simulink model "clrrtsf"  (R2020a)
settings: Solver=FixedStepAuto  StartTime=0.0  StopTime=inf  FixedStep=0.2  RelTol=1e-3
model workspace (MAT data in the model file):
  IC_theta0 = Simulink.Signal
  IC_theta0.DataType = 'auto'
  IC_theta0.Dimensions = -1
  IC_theta0.DimensionsMode = 'auto'
  IC_theta0.Complexity = 'auto'
  IC_theta0.SampleTime = -1
  IC_theta0.SamplingMode = 'auto'
  IC_theta0.InitialValue = '0'
  IC_x0 = Simulink.Signal
  IC_x0.DataType = 'auto'
  IC_x0.Dimensions = -1
  IC_x0.DimensionsMode = 'auto'
  IC_x0.Complexity = 'auto'
  IC_x0.SampleTime = -1
  IC_x0.SamplingMode = 'auto'
  IC_x0.InitialValue = '0'
  IC_x1 = Simulink.Signal
  IC_x1.DataType = 'auto'
  IC_x1.Dimensions = -1
  IC_x1.DimensionsMode = 'auto'
  IC_x1.Complexity = 'auto'
  IC_x1.SampleTime = -1
  IC_x1.SamplingMode = 'auto'
  IC_x1.InitialValue = '0'
  IC_y0 = Simulink.Signal
  IC_y0.DataType = 'auto'
  IC_y0.Dimensions = -1
  IC_y0.DimensionsMode = 'auto'
  IC_y0.Complexity = 'auto'
  IC_y0.SampleTime = -1
  IC_y0.SamplingMode = 'auto'
  IC_y1 = Simulink.Signal
  IC_y1.DataType = 'auto'
  IC_y1.Dimensions = -1
  IC_y1.DimensionsMode = 'auto'
  IC_y1.Complexity = 'auto'
  IC_y1.SampleTime = -1
  IC_y1.SamplingMode = 'auto'
  IC_y1.InitialValue = '0'
  contsim_time = Simulink.Signal
  contsim_time.DataType = 'double'
  contsim_time.Dimensions = [1 1]
  contsim_time.DimensionsMode = 'auto'
  contsim_time.Complexity = 'real'
  contsim_time.SampleTime = -1
  contsim_time.SamplingMode = 'auto'
  indicator = Simulink.Signal
  indicator.DataType = 'double'
  indicator.Dimensions = [1 4]
  indicator.DimensionsMode = 'auto'
  indicator.Complexity = 'real'
  indicator.SampleTime = -1
  indicator.SamplingMode = 'auto'
  indicator.InitialValue = '[0 0]'
  ip = Simulink.Signal
  ip.DataType = 'double'
  ip.Dimensions = [1 2]
  ip.DimensionsMode = 'auto'
  ip.Complexity = 'real'
  ip.SampleTime = -1
  ip.SamplingMode = 'auto'
  szxx1 = Simulink.Signal
  szxx1.DataType = 'double'
  szxx1.Dimensions = [1 1]
  szxx1.DimensionsMode = 'auto'
  szxx1.Complexity = 'real'
  szxx1.SampleTime = -1
  szxx1.SamplingMode = 'auto'
  szxx1.InitialValue = '0'
values from neighbouring files (symbols this model uses):
  indsimtime = 150    [clrrtsf_Initializ.m]
  L_0b = 0.48    [clrrtsf_Initializ.m]    (also in clrrtsolutionplot.m)
  L_0f = 3.8    [clrrtsf_Initializ.m]    (also in clrrtsolutionplot.m)
  L_1f = 7.21    [clrrtsf_Initializ.m]    (also in clrrtsolutionplot.m)
  LD = 10    [clrrtsf_Initializ.m]
  pinit = [80 160 pi 0]    [clrrtsf_Initializ.m]
  tn = zeros(N,14)    [clrrtsf_Initializ.m]    (also in clrrtsolutionplot.m = out.tree)
  veh_path = zeros(indsimtime,6)    [clrrtsf_Initializ.m]
  veh_path_col = zeros(indsimtime,6,N)    [clrrtsf_Initializ.m]
  xx = [-50:0.5:50]'    [clrrtsf_Initializ.m]
  yy = [-50:0.5:50]'    [clrrtsf_Initializ.m]
  Zf = griddata(x,y,znew,xnewt,ynewt)    [clrrtsf_Initializ.m]
  Zr = griddata(x,y,znewr,xnewt,ynewt)    [clrrtsf_Initializ.m]
undefined symbols (not defined in the file or in its folder): DiscIntNeverNeededParam, IC_theta1
libraries: simulink x1
(part 1 of 2)
settings Model: PauseTimes=0  OrderedModelArguments=off  Creator=giridhar  LastModifiedBy=giridhar
settings SolverCC: AlgebraicLoopSolver=LineSearch  MinimalZcImpactIntegration=on
settings DebuggingCC: ReadBeforeWriteMsg=DisableAll  WriteAfterWriteMsg=DisableAll  WriteAfterReadMsg=DisableAll  MultiTaskDSMMsg=none  SFUnusedDataAndEventsDiag=none  UnderSpecifiedDimensionMsg=warning
settings ModelReferenceCC: UpdateModelReferenceTargets=IfOutOfDate
settings SFSimCC: SFSimEcho=off

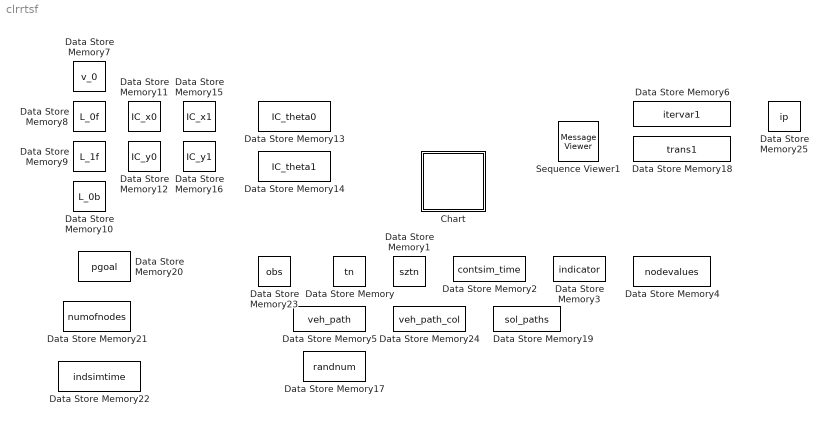
== system clrrtsf ==
  Chart : Stateflow chart  TreatAsAtomicUnit=on
  Data Store Memory : DataStoreMemory  DataStoreName=tn  ReadBeforeWriteMsg=warning  WriteAfterWriteMsg=warning  WriteAfterReadMsg=warning  InitialValue=tn  VectorParams1D=off  ShowAdditionalParam=off  OutDataTypeStr=double
  Data Store Memory1 : DataStoreMemory  DataStoreName=sztn  ReadBeforeWriteMsg=warning  WriteAfterWriteMsg=warning  WriteAfterReadMsg=warning  InitialValue=sztn  ShowAdditionalParam=off  OutDataTypeStr=double
  Data Store Memory10 : DataStoreMemory  DataStoreName=L_0b  ReadBeforeWriteMsg=warning  WriteAfterWriteMsg=warning  WriteAfterReadMsg=warning  InitialValue=0.48  VectorParams1D=off  ShowAdditionalParam=off  OutDataTypeStr=double  Dimensions=[1 1]
  Data Store Memory11 : DataStoreMemory  DataStoreName=IC_x0  ReadBeforeWriteMsg=warning  WriteAfterWriteMsg=warning  WriteAfterReadMsg=warning  VectorParams1D=off  ShowAdditionalParam=off  OutDataTypeStr=double  Dimensions=[1 1]
  Data Store Memory12 : DataStoreMemory  DataStoreName=IC_y0  ReadBeforeWriteMsg=warning  WriteAfterWriteMsg=warning  WriteAfterReadMsg=warning  VectorParams1D=off  ShowAdditionalParam=off  OutDataTypeStr=double  Dimensions=[1 1]
  Data Store Memory13 : DataStoreMemory  DataStoreName=IC_theta0  ReadBeforeWriteMsg=warning  WriteAfterWriteMsg=warning  WriteAfterReadMsg=warning  VectorParams1D=off  ShowAdditionalParam=off  OutDataTypeStr=double  Dimensions=[1 1]
  Data Store Memory14 : DataStoreMemory  DataStoreName=IC_theta1  ReadBeforeWriteMsg=warning  WriteAfterWriteMsg=warning  WriteAfterReadMsg=warning  VectorParams1D=off  ShowAdditionalParam=off  OutDataTypeStr=double  Dimensions=[1 1]
  Data Store Memory15 : DataStoreMemory  DataStoreName=IC_x1  ReadBeforeWriteMsg=warning  WriteAfterWriteMsg=warning  WriteAfterReadMsg=warning  VectorParams1D=off  ShowAdditionalParam=off  OutDataTypeStr=double  Dimensions=[1 1]  StateMustResolveToSignalObject=on
  Data Store Memory16 : DataStoreMemory  DataStoreName=IC_y1  ReadBeforeWriteMsg=warning  WriteAfterWriteMsg=warning  WriteAfterReadMsg=warning  VectorParams1D=off  ShowAdditionalParam=off  OutDataTypeStr=double  Dimensions=[1 1]  StateMustResolveToSignalObject=on
  Data Store Memory17 : DataStoreMemory  DataStoreName=randnum  ReadBeforeWriteMsg=warning  WriteAfterWriteMsg=warning  WriteAfterReadMsg=warning  InitialValue=randnum  ShowAdditionalParam=off  OutDataTypeStr=double
  Data Store Memory18 : DataStoreMemory  DataStoreName=trans1  ReadBeforeWriteMsg=warning  WriteAfterWriteMsg=warning  WriteAfterReadMsg=warning  VectorParams1D=off  ShowAdditionalParam=off  OutDataTypeStr=double
  Data Store Memory19 : DataStoreMemory  DataStoreName=sol_paths  ReadBeforeWriteMsg=warning  WriteAfterWriteMsg=warning  WriteAfterReadMsg=warning  ShowAdditionalParam=off
  Data Store Memory2 : DataStoreMemory  DataStoreName=contsim_time  ReadBeforeWriteMsg=warning  WriteAfterWriteMsg=warning  WriteAfterReadMsg=warning  VectorParams1D=off  ShowAdditionalParam=off  OutDataTypeStr=double  Dimensions=[1 1]  StateMustResolveToSignalObject=on
  Data Store Memory20 : DataStoreMemory  DataStoreName=pgoal  ReadBeforeWriteMsg=warning  WriteAfterWriteMsg=warning  WriteAfterReadMsg=warning  InitialValue=pgoal  VectorParams1D=off  ShowAdditionalParam=off  OutDataTypeStr=double
  Data Store Memory21 : DataStoreMemory  DataStoreName=numofnodes  ReadBeforeWriteMsg=warning  WriteAfterWriteMsg=warning  WriteAfterReadMsg=warning  InitialValue=numofnodes  VectorParams1D=off  ShowAdditionalParam=off  OutDataTypeStr=double
  Data Store Memory22 : DataStoreMemory  DataStoreName=indsimtime  ReadBeforeWriteMsg=warning  WriteAfterWriteMsg=warning  WriteAfterReadMsg=warning  InitialValue=indsimtime  ShowAdditionalParam=off  OutDataTypeStr=double
  Data Store Memory23 : DataStoreMemory  DataStoreName=obs  ReadBeforeWriteMsg=warning  WriteAfterWriteMsg=warning  WriteAfterReadMsg=warning  InitialValue=obs  VectorParams1D=off  ShowAdditionalParam=off  OutDataTypeStr=double
  Data Store Memory24 : DataStoreMemory  DataStoreName=veh_path_col  ReadBeforeWriteMsg=warning  WriteAfterWriteMsg=warning  WriteAfterReadMsg=warning  InitialValue=veh_path_col  VectorParams1D=off  ShowAdditionalParam=off  OutDataTypeStr=double
  Data Store Memory25 : DataStoreMemory  DataStoreName=ip  ReadBeforeWriteMsg=warning  WriteAfterWriteMsg=warning  WriteAfterReadMsg=warning  InitialValue=[0 0]  VectorParams1D=off  ShowAdditionalParam=off  OutDataTypeStr=double  Dimensions=[1 2]  StateMustResolveToSignalObject=on
  Data Store Memory3 : DataStoreMemory  DataStoreName=indicator  ReadBeforeWriteMsg=warning  WriteAfterWriteMsg=warning  WriteAfterReadMsg=warning  InitialValue=[0 0 0 0]  VectorParams1D=off  ShowAdditionalParam=off  OutDataTypeStr=double
  Data Store Memory4 : DataStoreMemory  DataStoreName=nodevalues  ReadBeforeWriteMsg=warning  WriteAfterWriteMsg=warning  WriteAfterReadMsg=warning  InitialValue=[0 0 0 0 0 0 0 0]  VectorParams1D=off  ShowAdditionalParam=off  OutDataTypeStr=double  Dimensions=[1 8]
  Data Store Memory5 : DataStoreMemory  DataStoreName=veh_path  ReadBeforeWriteMsg=warning  WriteAfterWriteMsg=warning  WriteAfterReadMsg=warning  InitialValue=veh_path  VectorParams1D=off  ShowAdditionalParam=off  OutDataTypeStr=double
  Data Store Memory6 : DataStoreMemory  DataStoreName=itervar1  ReadBeforeWriteMsg=warning  WriteAfterWriteMsg=warning  WriteAfterReadMsg=warning  VectorParams1D=off  ShowAdditionalParam=off  OutDataTypeStr=double
  Data Store Memory7 : DataStoreMemory  DataStoreName=v_0  ReadBeforeWriteMsg=warning  WriteAfterWriteMsg=warning  WriteAfterReadMsg=warning  InitialValue=v_0  VectorParams1D=off  ShowAdditionalParam=off  OutDataTypeStr=double  Dimensions=[1 1]
  Data Store Memory8 : DataStoreMemory  DataStoreName=L_0f  ReadBeforeWriteMsg=warning  WriteAfterWriteMsg=warning  WriteAfterReadMsg=warning  InitialValue=3.8  VectorParams1D=off  ShowAdditionalParam=off  OutDataTypeStr=double  Dimensions=[1 1]
  Data Store Memory9 : DataStoreMemory  DataStoreName=L_1f  ReadBeforeWriteMsg=warning  WriteAfterWriteMsg=warning  WriteAfterReadMsg=warning  InitialValue=7.21  VectorParams1D=off  ShowAdditionalParam=off  OutDataTypeStr=double  Dimensions=[1 1]
  Sequence Viewer1 : MessageViewer  History=1000  SavedRootId=#

== system clrrtsf/Chart/costcalculation.costcal ==
  i : Inport  OutDataTypeStr=double  PortDimensions=[1 1]
  f : TriggerPort  TriggerType=function-call  VariantControl=(inherit)
      settings: CopyFcn=Stateflow.SLINSF.SimulinkMan.removeBlockPreDeleteFcn  PreDeleteFcn=Stateflow.SLINSF.SimulinkMan.unsafePredeleteFcn
  Add : Sum
  Assignment5 : Assignment  NumberOfDimensions=2  DiagnosticForDimensions=Warning  IndexOptions=Index vector (port),Index vector (dialog)  Indices=1,1  OutputSizes=1,1
  Constant : Constant
  Data Store Read : DataStoreRead  DataStoreName=veh_path
  Data Store Read1 : DataStoreRead  DataStoreName=tn  DataStoreElements=tn(:,6)
  Data Store Write : DataStoreWrite  DataStoreName=tn  DataStoreElements=tn(:,6)
  MATLAB Function : MATLAB Function  TreatAsAtomicUnit=on
  wires:
  Data Store Read/1 -> MATLAB Function/1(veh_path)
  MATLAB Function/1(costt) -> Assignment5/2
  Data Store Read1/1 -> Assignment5/1
  Assignment5/1 -> Data Store Write/1
  i/1 -> Add/1
  Add/1 -> Assignment5/3
  Constant/1 -> Add/2

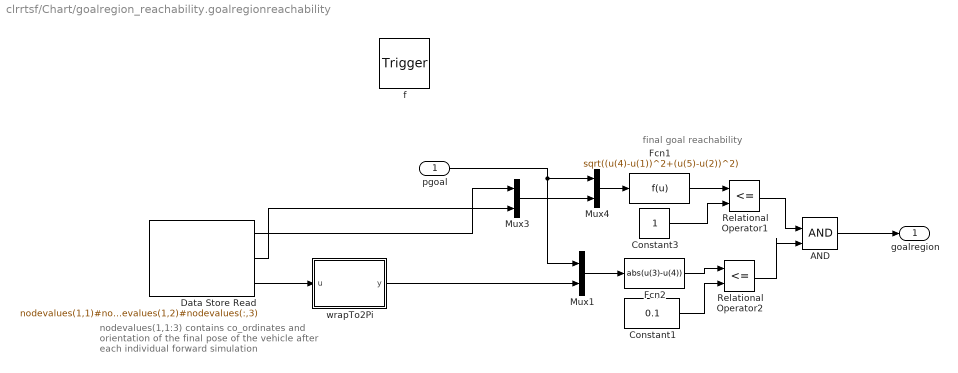
== system clrrtsf/Chart/goalregion_reachability.goalregionreachability ==
  note: nodevalues(1,1:3) contains co_ordinates
      | and orientation of the final pose of the
      | vehicle after each individual forward simulation
  note: final goal reachability
  pgoal : Inport  OutDataTypeStr=double  PortDimensions=[1 3]
  f : TriggerPort  TriggerType=function-call  VariantControl=(inherit)
      settings: CopyFcn=Stateflow.SLINSF.SimulinkMan.removeBlockPreDeleteFcn  PreDeleteFcn=Stateflow.SLINSF.SimulinkMan.unsafePredeleteFcn
  AND : Logic  IconShape=distinctive  AllPortsSameDT=off  OutDataTypeStr=boolean
  Constant1 : Constant  Value=0.1
  Constant3 : Constant
  Data Store Read : DataStoreRead  DataStoreName=nodevalues  DataStoreElements=nodevalues(1,1)#nodevalues(1,2)#nodevalues(:,3)
  Fcn1 : Fcn  Expr=sqrt((u(4)-u(1))^2+(u(5)-u(2))^2)
  Fcn2 : Fcn  Expr=abs(u(3)-u(4))
  Mux1 : Mux  Inputs=2
  Mux3 : Mux  Inputs=2
  Mux4 : Mux  Inputs=2
  Relational Operator1 : RelationalOperator  Operator=<=  OutDataTypeStr=boolean  RndMeth=Simplest
  Relational Operator2 : RelationalOperator  Operator=<=  OutDataTypeStr=boolean  RndMeth=Simplest
  wrapTo2Pi : MATLAB Function  TreatAsAtomicUnit=on
  goalregion : Outport
  wires:
  Constant1/1 -> Relational Operator2/2
  Relational Operator2/1 -> AND/2
  Mux1/1 -> Fcn2/1
  pgoal/1 -> Mux4/1, Mux1/1
  Mux3/1 -> Mux4/2
  Fcn2/1 -> Relational Operator2/1
  Constant3/1 -> Relational Operator1/2
  Fcn1/1 -> Relational Operator1/1
  Mux4/1 -> Fcn1/1
  Relational Operator1/1 -> AND/1
  Data Store Read/1 -> Mux3/1
  Data Store Read/2 -> Mux3/2
  Data Store Read/3 -> wrapTo2Pi/1(u)
  AND/1 -> goalregion/1
  wrapTo2Pi/1(y) -> Mux1/2

== system clrrtsf/Chart/output_to_workspace.output1wpace ==
  note: output to matlab workspace, all the details related to planning tree
      |  which were stored in the datastore "tn"
  note: output to matlab workspace, all the path co_ordinates and orientationof vehicle
      |  which were stored in the datastore "veh_path_col"
  f : TriggerPort  TriggerType=function-call  VariantControl=(inherit)
      settings: CopyFcn=Stateflow.SLINSF.SimulinkMan.removeBlockPreDeleteFcn  PreDeleteFcn=Stateflow.SLINSF.SimulinkMan.unsafePredeleteFcn
  Data Store Read : DataStoreRead  DataStoreName=tn  DataStoreElements=tn(:,:)
  Data Store Read1 : DataStoreRead  DataStoreName=veh_path_col  DataStoreElements=veh_path_col(:,1:4,:)
  To Workspace : ToWorkspace  VariableName=veh_path_col  SampleTime=-1
  To Workspace1 : ToWorkspace  VariableName=tree  SampleTime=-1
  wires:
  Data Store Read/1 -> To Workspace1/1
  Data Store Read1/1 -> To Workspace/1

== system clrrtsf/Chart/propagateorForwardsimulationstage.propagate ==
  note: subsystem to update
      | current start point node
      | and resets variables
      |  "itervar1" and "trans1"
  note: tractor longitudinal velocity
  note: gp is the intermediate goal point for the current
      | forward simulation, it can be a random sample
      | or a goal sample
  note: Nn_ is the node number of current start point, selected
      | based on the nearest neighbour or cheapest neighbour strategy
      | is uded to index into tree to find respective co-ordinates
  v_0 : Inport  OutDataTypeStr=double  PortDimensions=1
  gp : Inport  Port=2  OutMin=1  OutMax=2  OutDataTypeStr=double  PortDimensions=[1 3]
  Nn_ : Inport  Port=3  OutDataTypeStr=double  PortDimensions=1
  g : TriggerPort  TriggerType=function-call  VariantControl=(inherit)  SampleTime=0.2
      settings: CopyFcn=Stateflow.SLINSF.SimulinkMan.removeBlockPreDeleteFcn  PreDeleteFcn=Stateflow.SLINSF.SimulinkMan.unsafePredeleteFcn
  Data Store Read : DataStoreRead  DataStoreName=itervar1
  Delay : Delay  DelayLength=1
  Enabled Subsystem : Subsystem  TreatAsAtomicUnit=on
  Resettable Subsystem : Subsystem  Priority=1  TreatAsAtomicUnit=on
  Subsystem : Subsystem  Priority=2
  wires:
  gp/1 -> Subsystem/2(gp), Resettable Subsystem/2(gp)
  v_0/1 -> Resettable Subsystem/1(v_0)
  Nn_/1 -> Resettable Subsystem/3(Nn_), Enabled Subsystem/1(Nn_)
  Data Store Read/1 -> Subsystem/Enable, Subsystem/1(In1), Delay/1
  Delay/1 -> Enabled Subsystem/Enable, Resettable Subsystem/Reset

== system clrrtsf/Chart/stage1.f ==
  note: nearest neighbour
  sr : Inport  OutDataTypeStr=double  PortDimensions=[1 2]
  i : Inport  Port=2  OutDataTypeStr=double  PortDimensions=1
  f : TriggerPort  TriggerType=function-call  VariantControl=(inherit)  SampleTime=0.2
      settings: CopyFcn=Stateflow.SLINSF.SimulinkMan.removeBlockPreDeleteFcn  PreDeleteFcn=Stateflow.SLINSF.SimulinkMan.unsafePredeleteFcn
  For Iterator Subsystem : Subsystem  TreatAsAtomicUnit=on
  Nn : Outport  OutDataTypeStr=double
  wires:
  sr/1 -> For Iterator Subsystem/1(sr)
  For Iterator Subsystem/1(Nn) -> Nn/1
  i/1 -> For Iterator Subsystem/2(i)

== system clrrtsf/Chart/stage1.f_ ==
  note: cheapest neighbour
  note: random sample
  sr : Inport  OutDataTypeStr=double  PortDimensions=[1 2]
  i : Inport  Port=2  OutDataTypeStr=double  PortDimensions=1
  f : TriggerPort  TriggerType=function-call  VariantControl=(inherit)  SampleTime=0.2
      settings: CopyFcn=Stateflow.SLINSF.SimulinkMan.removeBlockPreDeleteFcn  PreDeleteFcn=Stateflow.SLINSF.SimulinkMan.unsafePredeleteFcn
  For Iterator Subsystem : Subsystem  TreatAsAtomicUnit=on
  Nn : Outport  OutDataTypeStr=double
  wires:
  sr/1 -> For Iterator Subsystem/1(sr)
  For Iterator Subsystem/1(Nn) -> Nn/1
  i/1 -> For Iterator Subsystem/2(i)

== system clrrtsf/Chart/stopsimulation ==
  Action Port : ActionPort
      settings: CopyFcn=Stateflow.SLINSF.SimulinkMan.removeBlockPreDeleteFcn  PreDeleteFcn=Stateflow.SLINSF.SimulinkMan.unsafePredeleteFcn
  Constant : Constant
  Stop Simulation : Stop
  wires:
  Constant/1 -> Stop Simulation/1

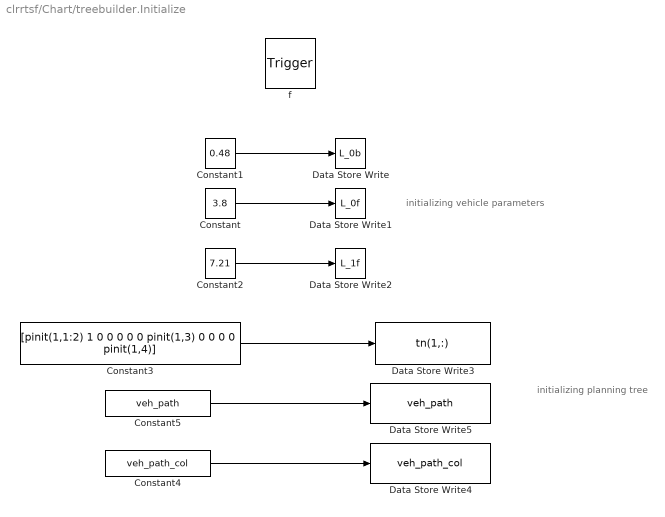
== system clrrtsf/Chart/treebuilder.Initialize ==
  note: initializing vehicle parameters
  note: initializing planning tree
  f : TriggerPort  TriggerType=function-call  VariantControl=(inherit)
      settings: CopyFcn=Stateflow.SLINSF.SimulinkMan.removeBlockPreDeleteFcn  PreDeleteFcn=Stateflow.SLINSF.SimulinkMan.unsafePredeleteFcn
  Constant : Constant  Value=3.8  VectorParams1D=off
  Constant1 : Constant  Value=0.48  VectorParams1D=off
  Constant2 : Constant  Value=7.21  VectorParams1D=off
  Constant3 : Constant  Value=[pinit(1,1:2) 1 0 0 0 0 0 pinit(1,3) 0 0 0 0 pinit(1,4)]  VectorParams1D=off
  Constant4 : Constant  Value=veh_path_col  VectorParams1D=off
  Constant5 : Constant  Value=veh_path  VectorParams1D=off
  Data Store Write : DataStoreWrite  DataStoreName=L_0b
  Data Store Write1 : DataStoreWrite  DataStoreName=L_0f
  Data Store Write2 : DataStoreWrite  DataStoreName=L_1f
  Data Store Write3 : DataStoreWrite  DataStoreName=tn  DataStoreElements=tn(1,:)
  Data Store Write4 : DataStoreWrite  DataStoreName=veh_path_col
  Data Store Write5 : DataStoreWrite  DataStoreName=veh_path
  wires:
  Constant/1 -> Data Store Write1/1
  Constant2/1 -> Data Store Write2/1
  Constant1/1 -> Data Store Write/1
  Constant3/1 -> Data Store Write3/1
  Constant4/1 -> Data Store Write4/1
  Constant5/1 -> Data Store Write5/1

== system clrrtsf/Chart/treebuilder.cumilativecost ==
  "i " : Inport  OutDataTypeStr=double  PortDimensions=[1 1]
  f : TriggerPort  TriggerType=function-call  VariantControl=(inherit)
      settings: CopyFcn=Stateflow.SLINSF.SimulinkMan.removeBlockPreDeleteFcn  PreDeleteFcn=Stateflow.SLINSF.SimulinkMan.unsafePredeleteFcn
  Assignment6 : Assignment  NumberOfDimensions=2  DiagnosticForDimensions=Warning  IndexOptions=Index vector (port),Index vector (dialog)  Indices=1,1  OutputSizes=1,1
  Data Store Read : DataStoreRead  DataStoreName=tn
  Data Store Read1 : DataStoreRead  DataStoreName=tn  DataStoreElements=tn(:,7)
  Data Store Write : DataStoreWrite  DataStoreName=tn  DataStoreElements=tn(:,7)
  MATLAB Function : MATLAB Function  TreatAsAtomicUnit=on
  wires:
  Data Store Read/1 -> MATLAB Function/1(tn)
  Data Store Read1/1 -> Assignment6/1
  "i "/1 -> Assignment6/3, MATLAB Function/2(i)
  MATLAB Function/1(totallen) -> Assignment6/2
  Assignment6/1 -> Data Store Write/1

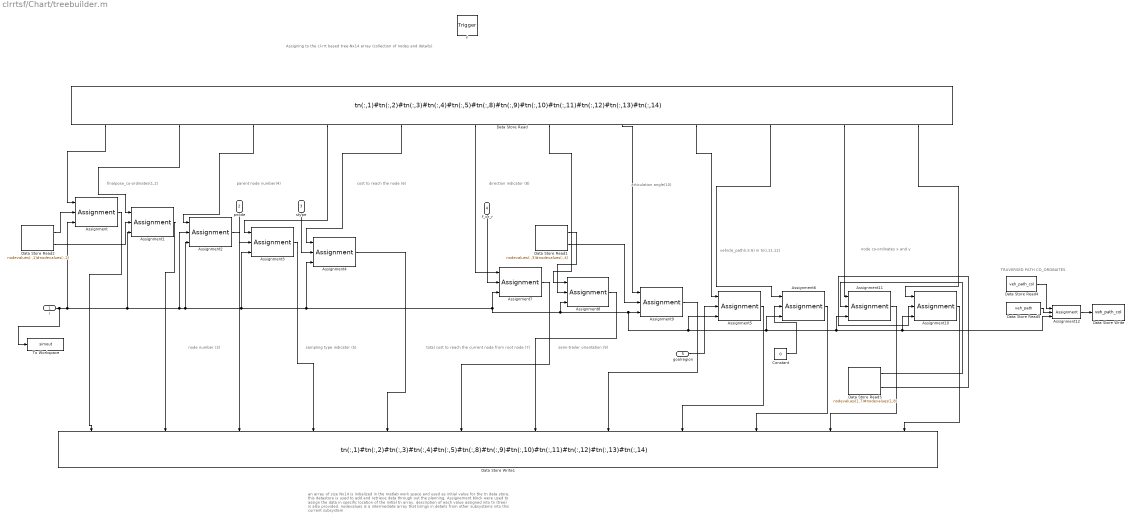
== system clrrtsf/Chart/treebuilder.m ==
  note: an array of size Nx14 is initialized in the matlab work space and used as initial value for the tn data store,
      | this datastore is used to add and retrieve data through out the planning, Assignement block were used to
      | assign the data in specific location of the initial tn array, description of each value assigned into tn (tree) is
      | also provided. nodevalues is a intermediate array that brings in details from other subsystems into this current subsystem
  note: TRAVERSED PATH CO_ORDINATES
  note: node co-ordinates x and y
  note: finalpose_co-ordinates(1,2)
  note: node number (3)
  note: parent node number(4)
  note: sampling type indicator (5)
  note: cost to reach the node (6)
  note: total cost to reach the
      | current node from root node (7)
  note: direction indicator (8)
  note: vehicle_path(i,5:6) in tn(i,11,12)
  note: Assigning to the cl-rrt based tree-Nx14 array (collection of nodes and details)
  note: semi-trailer orientation (9)
  note: articulation angle(10)
  i : Inport  OutDataTypeStr=double  PortDimensions=1
  pnode : Inport  Port=2  OutDataTypeStr=double  PortDimensions=1
  stype : Inport  Port=3  OutDataTypeStr=double  PortDimensions=[1 1]
  f_or_r : Inport  Port=4  OutDataTypeStr=double  PortDimensions=[1 1]
  goalregion : Inport  Port=5  OutDataTypeStr=double  PortDimensions=1
  f : TriggerPort  TriggerType=function-call  VariantControl=(inherit)
      settings: CopyFcn=Stateflow.SLINSF.SimulinkMan.removeBlockPreDeleteFcn  PreDeleteFcn=Stateflow.SLINSF.SimulinkMan.unsafePredeleteFcn
  Assignment{,1..11} (12 alike) : Assignment  NumberOfDimensions=2  DiagnosticForDimensions=Warning  IndexOptions=Index vector (port),Index vector (dialog)  Indices=1,1  OutputSizes=1,1
  Assignment12 : Assignment  NumberOfDimensions=3  DiagnosticForDimensions=Warning  IndexOptions=Assign all,Assign all,Index vector (port)  Indices=1,1,1  OutputSizes=1,1,1
  Constant : Constant  Value=0
  Data Store Read : DataStoreRead  DataStoreName=tn  DataStoreElements=tn(:,1)#tn(:,2)#tn(:,3)#tn(:,4)#tn(:,5)#tn(:,8)#tn(:,9)#tn(:,10)#tn(:,11)#tn(:,12)#tn(:,13)#tn(:,14)
  Data Store Read1 : DataStoreRead  DataStoreName=nodevalues  DataStoreElements=nodevalues(:,3)#nodevalues(:,4)
  Data Store Read2 : DataStoreRead  DataStoreName=nodevalues  DataStoreElements=nodevalues(:,1)#nodevalues(:,2)
  Data Store Read3 : DataStoreRead  DataStoreName=nodevalues  DataStoreElements=nodevalues(1,7)#nodevalues(1,8)
  Data Store Read4 : DataStoreRead  DataStoreName=veh_path_col
  Data Store Read5 : DataStoreRead  DataStoreName=veh_path
  Data Store Write : DataStoreWrite  DataStoreName=veh_path_col
  Data Store Write1 : DataStoreWrite  DataStoreName=tn  DataStoreElements=tn(:,1)#tn(:,2)#tn(:,3)#tn(:,4)#tn(:,5)#tn(:,8)#tn(:,9)#tn(:,10)#tn(:,11)#tn(:,12)#tn(:,13)#tn(:,14)
  To Workspace : ToWorkspace  VariableName=simout  SaveFormat=Timeseries  SampleTime=-1
  wires:
  stype/1 -> Assignment4/2
  f_or_r/1 -> Assignment7/2
  Assignment1/1 -> Data Store Write1/2
  pnode/1 -> Assignment3/2
  Data Store Read2/2 -> Assignment1/2
  Data Store Read2/1 -> Assignment/2
  Data Store Read/1 -> Assignment/1
  Data Store Read1/1 -> Assignment8/2
  i/1 -> To Workspace/1, Assignment2/3, Assignment8/3, Assignment5/3, Assignment12/3, Assignment10/3, Assignment11/3, Assignment6/3, Assignment9/3, Assignment7/3, Assignment4/3, Assignment3/3, Assignment2/2, Assignment1/3, Assignment/3
  Data Store Read1/2 -> Assignment9/2
  Data Store Read3/1 -> Assignment11/2
  Data Store Read3/2 -> Assignment10/2
  Constant/1 -> Assignment6/2
  goalregion/1 -> Assignment5/2
  Assignment/1 -> Data Store Write1/1
  Data Store Read/2 -> Assignment1/1
  Data Store Read/3 -> Assignment2/1
  Assignment2/1 -> Data Store Write1/3
  Assignment3/1 -> Data Store Write1/4
  Assignment4/1 -> Data Store Write1/5
  Data Store Read/4 -> Assignment3/1
  Data Store Read/5 -> Assignment4/1
  Data Store Read/6 -> Assignment7/1
  Assignment7/1 -> Data Store Write1/6
  Assignment8/1 -> Data Store Write1/7
  Data Store Read/7 -> Assignment8/1
  Data Store Read/8 -> Assignment9/1
  Assignment9/1 -> Data Store Write1/8
  Data Store Read/9 -> Assignment5/1
  Assignment5/1 -> Data Store Write1/9
  Data Store Read/10 -> Assignment6/1
  Assignment6/1 -> Data Store Write1/10
  Data Store Read/11 -> Assignment11/1
  Assignment11/1 -> Data Store Write1/11
  Data Store Read/12 -> Assignment10/1
  Assignment10/1 -> Data Store Write1/12
  Data Store Read4/1 -> Assignment12/1
  Data Store Read5/1 -> Assignment12/2
  Assignment12/1 -> Data Store Write/1

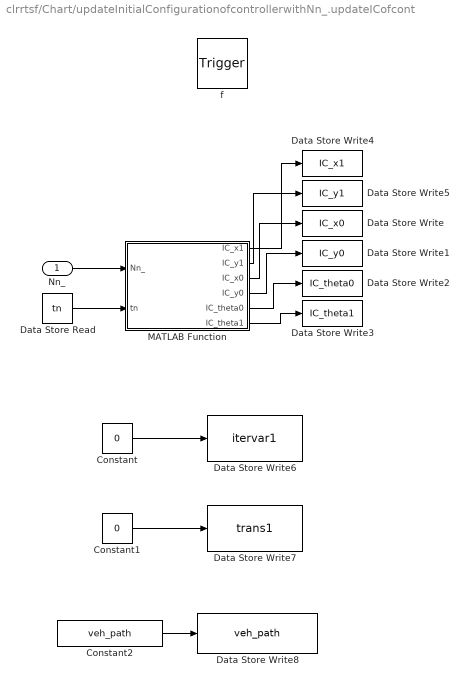
== system clrrtsf/Chart/updateInitialConfigurationofcontrollerwithNn_.updateICofcont ==
  Nn_ : Inport  OutDataTypeStr=double  PortDimensions=1
  f : TriggerPort  TriggerType=function-call  VariantControl=(inherit)
      settings: CopyFcn=Stateflow.SLINSF.SimulinkMan.removeBlockPreDeleteFcn  PreDeleteFcn=Stateflow.SLINSF.SimulinkMan.unsafePredeleteFcn
  Constant : Constant  Value=0
  Constant1 : Constant  Value=0
  Constant2 : Constant  Value=veh_path  VectorParams1D=off
  Data Store Read : DataStoreRead  DataStoreName=tn
  Data Store Write : DataStoreWrite  DataStoreName=IC_x0
  Data Store Write1 : DataStoreWrite  DataStoreName=IC_y0
  Data Store Write2 : DataStoreWrite  DataStoreName=IC_theta0
  Data Store Write3 : DataStoreWrite  DataStoreName=IC_theta1
  Data Store Write4 : DataStoreWrite  DataStoreName=IC_x1
  Data Store Write5 : DataStoreWrite  DataStoreName=IC_y1
  Data Store Write6 : DataStoreWrite  DataStoreName=itervar1
  Data Store Write7 : DataStoreWrite  DataStoreName=trans1
  Data Store Write8 : DataStoreWrite  DataStoreName=veh_path
  MATLAB Function : MATLAB Function  TreatAsAtomicUnit=on
  wires:
  Nn_/1 -> MATLAB Function/1(Nn_)
  Data Store Read/1 -> MATLAB Function/2(tn)
  MATLAB Function/6(IC_theta1) -> Data Store Write3/1
  MATLAB Function/5(IC_theta0) -> Data Store Write2/1
  MATLAB Function/4(IC_y0) -> Data Store Write1/1
  MATLAB Function/3(IC_x0) -> Data Store Write/1
  MATLAB Function/2(IC_y1) -> Data Store Write5/1
  MATLAB Function/1(IC_x1) -> Data Store Write4/1
  Constant/1 -> Data Store Write6/1
  Constant1/1 -> Data Store Write7/1
  Constant2/1 -> Data Store Write8/1

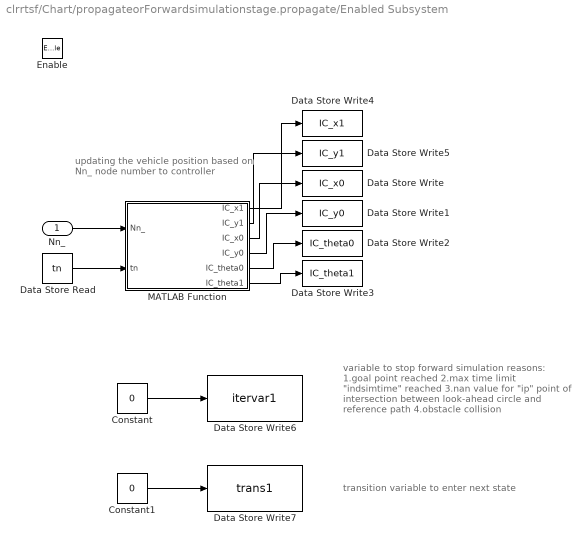
== system clrrtsf/Chart/propagateorForwardsimulationstage.propagate/Enabled Subsystem ==
  note: updating the vehicle position based on
      | Nn_ node number to controller
  note: variable to stop forward simulation
      | reasons:
      | 1.goal point reached
      | 2.max time limit "indsimtime" reached
      | 3.nan value for "ip" point of intersection
      |  between look-ahead circle and reference path
      | 4.obstacle collision
  note: transition variable to enter next state
  Nn_ : Inport  OutDataTypeStr=double  PortDimensions=1
  Enable : EnablePort  StatesWhenEnabling=reset
  Constant : Constant  Value=0
  Constant1 : Constant  Value=0
  Data Store Read : DataStoreRead  DataStoreName=tn
  Data Store Write : DataStoreWrite  DataStoreName=IC_x0
  Data Store Write1 : DataStoreWrite  DataStoreName=IC_y0
  Data Store Write2 : DataStoreWrite  DataStoreName=IC_theta0
  Data Store Write3 : DataStoreWrite  DataStoreName=IC_theta1
  Data Store Write4 : DataStoreWrite  DataStoreName=IC_x1
  Data Store Write5 : DataStoreWrite  DataStoreName=IC_y1
  Data Store Write6 : DataStoreWrite  DataStoreName=itervar1
  Data Store Write7 : DataStoreWrite  DataStoreName=trans1
  MATLAB Function : MATLAB Function  TreatAsAtomicUnit=on
  wires:
  Nn_/1 -> MATLAB Function/1(Nn_)
  Constant/1 -> Data Store Write6/1
  Constant1/1 -> Data Store Write7/1
  MATLAB Function/1(IC_x1) -> Data Store Write4/1
  Data Store Read/1 -> MATLAB Function/2(tn)
  MATLAB Function/2(IC_y1) -> Data Store Write5/1
  MATLAB Function/5(IC_theta0) -> Data Store Write2/1
  MATLAB Function/3(IC_x0) -> Data Store Write/1
  MATLAB Function/4(IC_y0) -> Data Store Write1/1
  MATLAB Function/6(IC_theta1) -> Data Store Write3/1

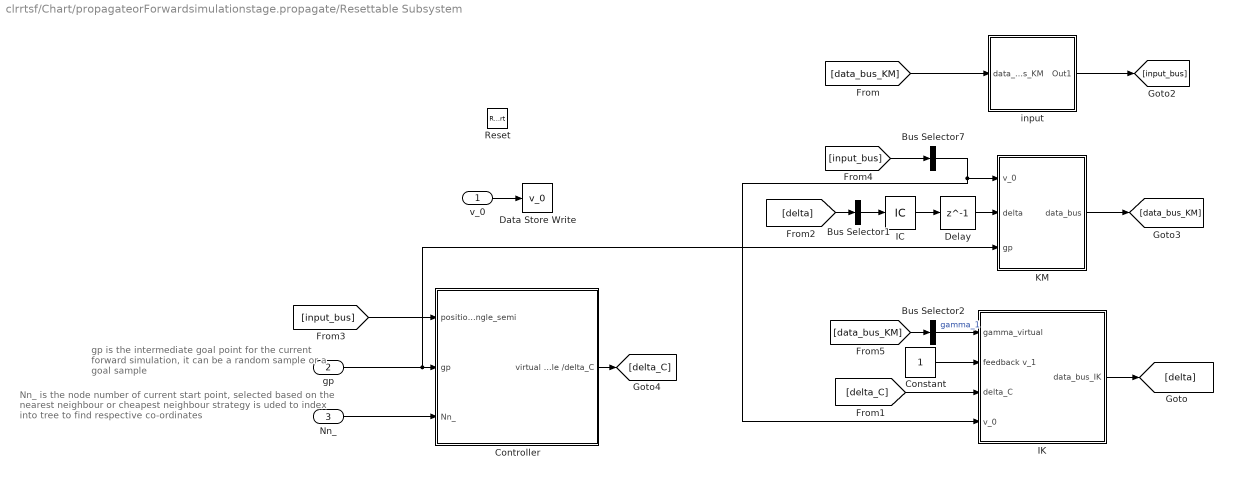
== system clrrtsf/Chart/propagateorForwardsimulationstage.propagate/Resettable Subsystem ==
  note: gp is the intermediate goal point for the current
      | forward simulation, it can be a random sample
      | or a goal sample
  note: Nn_ is the node number of current start point, selected
      | based on the nearest neighbour or cheapest neighbour strategy
      | is uded to index into tree to find respective co-ordinates
  v_0 : Inport  OutDataTypeStr=double  PortDimensions=1
  gp : Inport  Port=2  OutMin=1  OutMax=2  OutDataTypeStr=double  PortDimensions=[1 3]
  Nn_ : Inport  Port=3  OutDataTypeStr=double  PortDimensions=1
  Reset : ResetPort  DisableCoverage=on  ResetTriggerType=level  PropagateVarSize=During execution
  Bus Selector1 : BusSelector  OutputSignals=angle.steering_angle  OutputAsBus=on
  Bus Selector2 : BusSelector  OutputSignals=angle.articulation_angle  OutputAsBus=on
  Bus Selector7 : BusSelector  OutputSignals=u_0  OutputAsBus=on
  Constant : Constant
  Controller : Subsystem  TreatAsAtomicUnit=on
  Data Store Write : DataStoreWrite  DataStoreName=v_0
  Delay : Delay  DelayLength=1
  IC : InitialCondition  Value=0
  IK : Subsystem  SystemSampleTime=0.8
  KM : Subsystem  SystemSampleTime=0.8
  input : Subsystem
  wires:
  [data_bus_KM] -> Bus Selector2/1
  input/1(Out1) -> [input_bus]
  [delta_C] -> IK/3(delta_C)
  Bus Selector7/1 -> IK/4(v_0), KM/1(v_0)
  [delta] -> Bus Selector1/1
  Nn_/1 -> Controller/3(Nn_)
  Delay/1 -> KM/2(delta)
  Constant/1 -> IK/2(feedback v_1)
  IC/1 -> Delay/1
  KM/1(data_bus) -> [data_bus_KM]
  Controller/1(virtual steer angle /delta_C) -> [delta_C]
  Bus Selector2/1 -> IK/1(gamma_virtual)  "gamma_1"
  Bus Selector1/1 -> IC/1
  gp/1 -> Controller/2(gp), KM/3(gp)
  v_0/1 -> Data Store Write/1
  IK/1(data_bus_IK) -> [delta]
  [input_bus] -> Bus Selector7/1
  [data_bus_KM] -> input/1(data_bus_KM)
  [input_bus] -> Controller/1(positions_yawangle_semi)

== system clrrtsf/Chart/propagateorForwardsimulationstage.propagate/Subsystem ==
  note: transition variable  when 1,
      |  next state is entered
  In1 : Inport
  gp : Inport  Port=2
  Enable : EnablePort  StatesWhenEnabling=reset
  Subsystem : Subsystem  Priority=2
  Subsystem1 : Subsystem  Priority=1
  wires:
  In1/1 -> Subsystem/1(In1)
  gp/1 -> Subsystem1/1(gp)

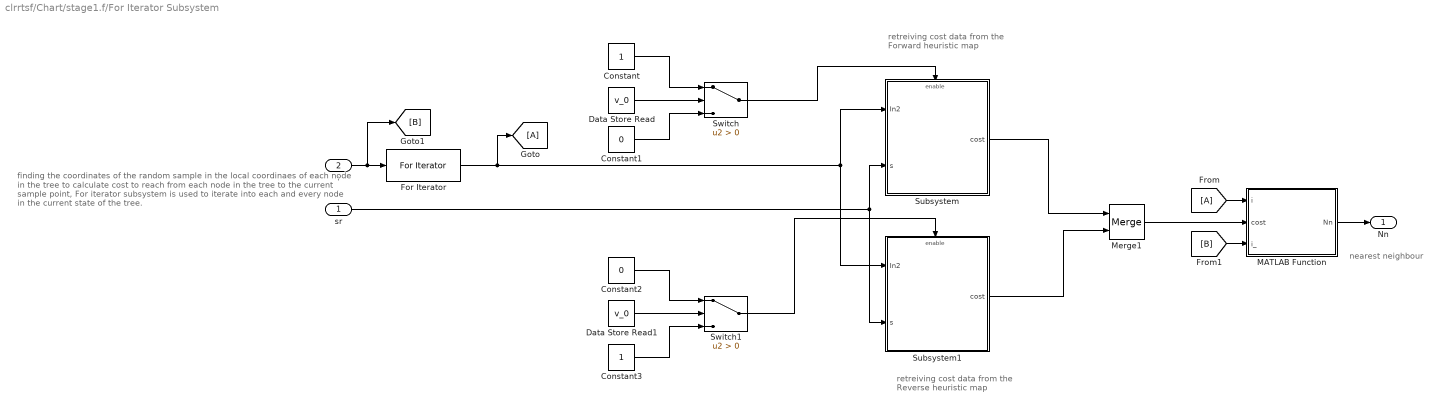
== system clrrtsf/Chart/stage1.f/For Iterator Subsystem ==
  note: nearest neighbour
  note: retreiving cost data from
      | the Forward heuristic map
  note: retreiving cost data from
      | the Reverse heuristic map
  note: finding the coordinates of the random sample in the local coordinaes
      |  of each node in the tree to calculate cost to reach from each node in
      | the tree to the current sample point, For iterator subsystem is used to iterate
      | into each and every node in the current state of the tree.
  sr : Inport  OutDataTypeStr=double  PortDimensions=[1 2]
  i : Inport  Port=2  OutDataTypeStr=double
  Constant : Constant
  Constant1 : Constant  Value=0
  Constant2 : Constant  Value=0
  Constant3 : Constant
  Data Store Read : DataStoreRead  DataStoreName=v_0
  Data Store Read1 : DataStoreRead  DataStoreName=v_0
  For Iterator : ForIterator  ResetStates=reset  IterationSource=external  IterationLimit=sztn  IterationVariableDataType=double
  MATLAB Function : MATLAB Function  TreatAsAtomicUnit=on
  Merge1 : Merge
  Subsystem : Subsystem
  Subsystem1 : Subsystem
  Switch : Switch  Criteria=u2 > Threshold
  Switch1 : Switch  Criteria=u2 > Threshold
  Nn : Outport  OutDataTypeStr=double  PortDimensions=[1 1]
  wires:
  For Iterator/1 -> [A], Subsystem/1(In2), Subsystem1/1(In2)
  sr/1 -> Subsystem/2(s), Subsystem1/2(s)
  Data Store Read/1 -> Switch/2
  Switch/1 -> Subsystem/Enable
  Constant/1 -> Switch/1
  Constant1/1 -> Switch/3
  Data Store Read1/1 -> Switch1/2
  Constant3/1 -> Switch1/3
  Constant2/1 -> Switch1/1
  Switch1/1 -> Subsystem1/Enable
  [A] -> MATLAB Function/1(i)
  Subsystem/1(cost) -> Merge1/1
  i/1 -> [B], For Iterator/1
  Subsystem1/1(cost) -> Merge1/2
  Merge1/1 -> MATLAB Function/2(cost)
  MATLAB Function/1(Nn) -> Nn/1
  [B] -> MATLAB Function/3(i_)

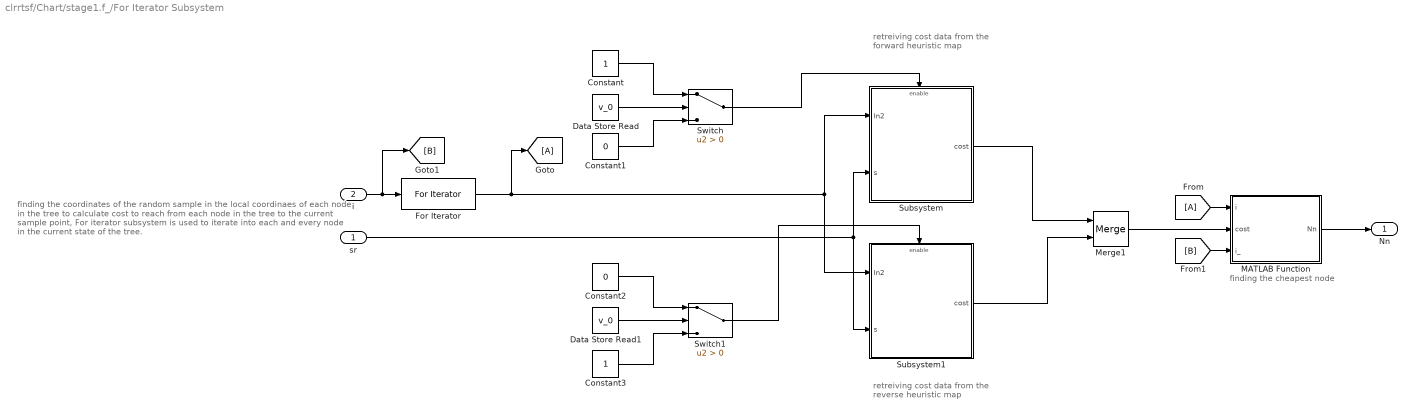
== system clrrtsf/Chart/stage1.f_/For Iterator Subsystem ==
  note: finding the cheapest node
  note: retreiving cost data from
      | the forward heuristic map
  note: finding the coordinates of the random sample in the local coordinaes
      |  of each node in the tree to calculate cost to reach from each node in
      | the tree to the current sample point, For iterator subsystem is used to iterate
      | into each and every node in the current state of the tree.
  note: retreiving cost data from
      | the reverse heuristic map
  sr : Inport  OutDataTypeStr=double  PortDimensions=[1 2]
  i : Inport  Port=2  OutDataTypeStr=double
  Constant : Constant
  Constant1 : Constant  Value=0
  Constant2 : Constant  Value=0
  Constant3 : Constant
  Data Store Read : DataStoreRead  DataStoreName=v_0
  Data Store Read1 : DataStoreRead  DataStoreName=v_0
  For Iterator : ForIterator  ResetStates=reset  IterationSource=external  IterationLimit=sztn  IterationVariableDataType=double
  MATLAB Function : MATLAB Function  TreatAsAtomicUnit=on
  Merge1 : Merge
  Subsystem : Subsystem
  Subsystem1 : Subsystem
  Switch : Switch  Criteria=u2 > Threshold
  Switch1 : Switch  Criteria=u2 > Threshold
  Nn : Outport  OutDataTypeStr=double  PortDimensions=[1 1]
  wires:
  [A] -> MATLAB Function/1(i)
  MATLAB Function/1(Nn) -> Nn/1
  Switch/1 -> Subsystem/Enable
  Data Store Read/1 -> Switch/2
  Constant3/1 -> Switch1/3
  Data Store Read1/1 -> Switch1/2
  Merge1/1 -> MATLAB Function/2(cost)
  Constant2/1 -> Switch1/1
  Constant1/1 -> Switch/3
  Constant/1 -> Switch/1
  Subsystem/1(cost) -> Merge1/1
  For Iterator/1 -> [A], Subsystem/1(In2), Subsystem1/1(In2)
  i/1 -> [B], For Iterator/1
  sr/1 -> Subsystem/2(s), Subsystem1/2(s)
  Subsystem1/1(cost) -> Merge1/2
  Switch1/1 -> Subsystem1/Enable
  [B] -> MATLAB Function/3(i_)

== system clrrtsf/Chart/propagateorForwardsimulationstage.propagate/Resettable Subsystem/Controller ==
  positions_yawangle_semi : Inport
  gp : Inport  Port=2
  Nn_ : Inport  Port=3
  Bus Selector1 : BusSelector  OutputSignals=yawangle_semi  OutputAsBus=on
  Bus Selector2 : BusSelector  OutputSignals=positions  OutputAsBus=on
  Differentiator/filter : Subsystem  mask{ts=13.5}
      mask prompts: ts "response_time"
      mask init:
      | c=(3*pi/ts)^2;
  Gain4 : Gain  Gain=-1
  distance to react1 : Saturate  UpperLimit=1  LowerLimit=-1
  purepursuit_contrroller : Subsystem
  virtual steer angle /delta_C : Outport  PortDimensions=[1,1]  VectorParamsAs1DForOutWhenUnconnected=off
  wires:
  Bus Selector1/1 -> purepursuit_contrroller/2(yawangle_semi)
  Differentiator/filter/1(Out1) -> virtual steer angle /delta_C/1
  Gain4/1 -> distance to react1/1
  Nn_/1 -> purepursuit_contrroller/4(Nn_)
  Bus Selector2/1 -> purepursuit_contrroller/1(driveaxle)  "driveaxle"
  distance to react1/1 -> Differentiator/filter/1(In1)
  gp/1 -> purepursuit_contrroller/3(gp)
  purepursuit_contrroller/1(steeringangle) -> Gain4/1
  positions_yawangle_semi/1 -> Bus Selector1/1, Bus Selector2/1

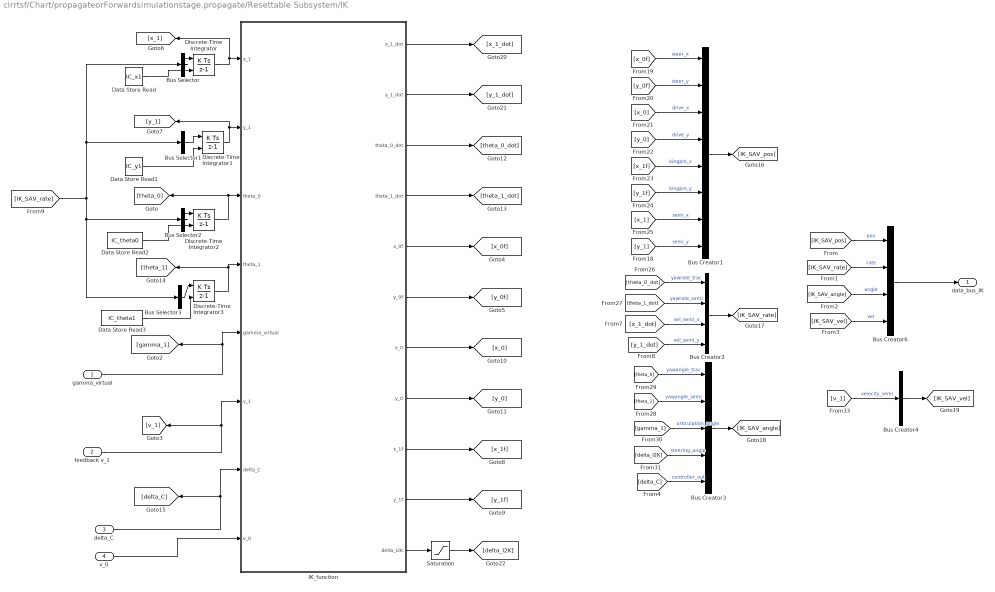
== system clrrtsf/Chart/propagateorForwardsimulationstage.propagate/Resettable Subsystem/IK ==
  gamma_virtual : Inport
  feedback v_1 : Inport  Port=2
  delta_C : Inport  Port=3
  v_0 : Inport  Port=4
  Bus Creator1 : BusCreator  Inputs=8
  Bus Creator2 : BusCreator  Inputs=4
  Bus Creator3 : BusCreator  Inputs=5
  Bus Creator4 : BusCreator  Inputs=1
  Bus Creator6 : BusCreator  Inputs=4
  Bus Selector : BusSelector  OutputSignals=vel_semi_x  OutputAsBus=on
  Bus Selector1 : BusSelector  OutputSignals=vel_semi_y  OutputAsBus=on
  Bus Selector2 : BusSelector  OutputSignals=yawrate_trac  OutputAsBus=on
  Bus Selector3 : BusSelector  OutputSignals=yawrate_semi  OutputAsBus=on
  Data Store Read : DataStoreRead  DataStoreName=IC_x1
  Data Store Read1 : DataStoreRead  DataStoreName=IC_y1
  Data Store Read2 : DataStoreRead  DataStoreName=IC_theta0
  Data Store Read3 : DataStoreRead  DataStoreName=IC_theta1
  Discrete-Time Integrator : DiscreteIntegrator  InitialConditionSource=external  InitialCondition=IC_x1  SampleTime=-1  ICPrevOutput=DiscIntNeverNeededParam  ICPrevScaledInput=DiscIntNeverNeededParam
  Discrete-Time Integrator1 : DiscreteIntegrator  InitialConditionSource=external  InitialCondition=IC_y1  SampleTime=-1  ICPrevOutput=DiscIntNeverNeededParam  ICPrevScaledInput=DiscIntNeverNeededParam
  Discrete-Time Integrator2 : DiscreteIntegrator  InitialConditionSource=external  InitialCondition=IC_theta0  SampleTime=-1  ICPrevOutput=DiscIntNeverNeededParam  ICPrevScaledInput=DiscIntNeverNeededParam
  Discrete-Time Integrator3 : DiscreteIntegrator  InitialConditionSource=external  InitialCondition=IC_theta1  SampleTime=-1  ICPrevOutput=DiscIntNeverNeededParam  ICPrevScaledInput=DiscIntNeverNeededParam
  IK_function : MATLAB Function  TreatAsAtomicUnit=on
  Saturation : Saturate  UpperLimit=0.7  LowerLimit=-0.7
  data_bus_IK : Outport  VectorParamsAs1DForOutWhenUnconnected=off
  wires:
  IK_function/7(x_0) -> [x_0]
  IK_function/8(y_0) -> [y_0]
  IK_function/1(x_1_dot) -> [x_1_dot]
  IK_function/3(theta_0_dot) -> [theta_0_dot]
  IK_function/4(theta_1_dot) -> [theta_1_dot]
  IK_function/10(y_1f) -> [y_1f]
  IK_function/9(x_1f) -> [x_1f]
  Discrete-Time Integrator/1 -> [x_1], IK_function/1(x_1)
  Discrete-Time Integrator1/1 -> [y_1], IK_function/2(y_1)
  gamma_virtual/1 -> [gamma_1], IK_function/5(gamma_virtual)
  IK_function/2(y_1_dot) -> [y_1_dot]
  delta_C/1 -> IK_function/7(delta_C), [delta_C]
  Discrete-Time Integrator3/1 -> IK_function/4(theta_1), [theta_1]
  IK_function/5(x_0f) -> [x_0f]
  IK_function/6(y_0f) -> [y_0f]
  [y_0f] -> Bus Creator1/2  "steer_y"
  [x_1f] -> Bus Creator1/5  "kingpin_x"
  Bus Creator6/1 -> data_bus_IK/1
  [v_1] -> Bus Creator4/1  "velocity_semi"
  [x_0] -> Bus Creator1/3  "drive_x"
  [y_1f] -> Bus Creator1/6  "kingpin_y"
  [x_0f] -> Bus Creator1/1  "steer_x"
  [y_0] -> Bus Creator1/4  "drive_y"
  Bus Creator3/1 -> [IK_SAV_angle]
  [theta_0_dot] -> Bus Creator2/1  "yawrate_trac"
  [theta_1_dot] -> Bus Creator2/2  "yawrate_semi"
  Discrete-Time Integrator2/1 -> [theta_0], IK_function/3(theta_0)
  [IK_SAV_rate] -> Bus Selector/1, Bus Selector1/1, Bus Selector3/1, Bus Selector2/1
  Bus Creator2/1 -> [IK_SAV_rate]
  Bus Creator1/1 -> [IK_SAV_pos]
  [delta_I2K] -> Bus Creator3/4  "steering_angle"
  [gamma_1] -> Bus Creator3/3  "articulation_angle"
  Bus Creator4/1 -> [IK_SAV_vel]
  [theta_1] -> Bus Creator3/2  "yawangle_semi"
  [IK_SAV_rate] -> Bus Creator6/2  "rate"
  [theta_0] -> Bus Creator3/1  "yawangle_trac"
  [IK_SAV_pos] -> Bus Creator6/1  "pos"
  [IK_SAV_angle] -> Bus Creator6/3  "angle"
  [IK_SAV_vel] -> Bus Creator6/4  "vel"
  Bus Selector3/1 -> Discrete-Time Integrator3/1
  Bus Selector2/1 -> Discrete-Time Integrator2/1
  Bus Selector/1 -> Discrete-Time Integrator/1
  Bus Selector1/1 -> Discrete-Time Integrator1/1
  [y_1_dot] -> Bus Creator2/4  "vel_semi_y"
  [x_1_dot] -> Bus Creator2/3  "vel_semi_x"
  IK_function/11(delta_I2K) -> Saturation/1
  [delta_C] -> Bus Creator3/5  "controller_out"
  feedback v_1/1 -> [v_1], IK_function/6(v_1)
  Saturation/1 -> [delta_I2K]
  [y_1] -> Bus Creator1/8  "semi_y"
  [x_1] -> Bus Creator1/7  "semi_x"
  Data Store Read3/1 -> Discrete-Time Integrator3/2
  Data Store Read2/1 -> Discrete-Time Integrator2/2
  Data Store Read1/1 -> Discrete-Time Integrator1/2
  Data Store Read/1 -> Discrete-Time Integrator/2
  v_0/1 -> IK_function/8(v_0)

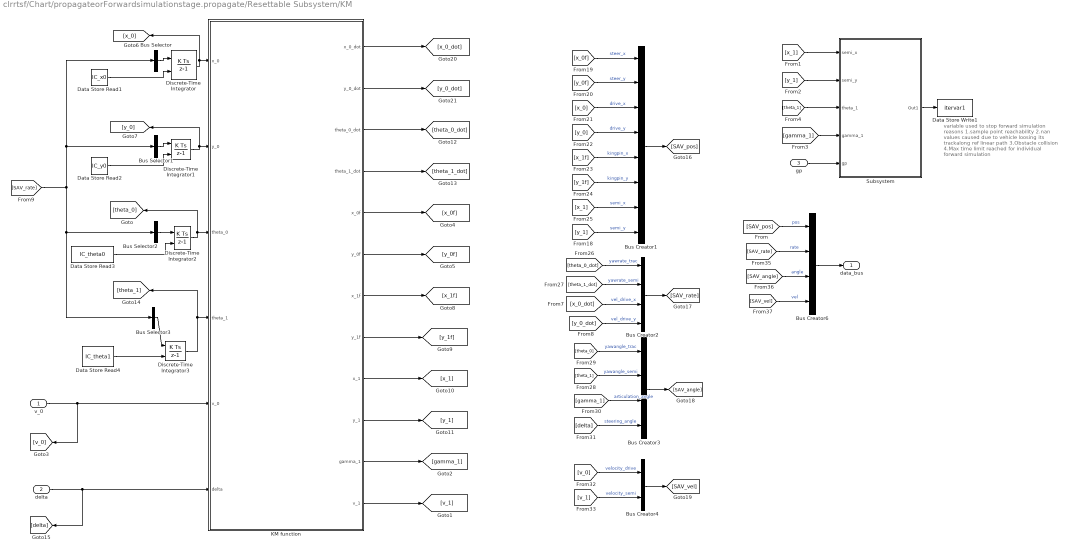
== system clrrtsf/Chart/propagateorForwardsimulationstage.propagate/Resettable Subsystem/KM ==
  note: variable used to stop forward simulation
      | reasons
      | 1.sample point reachability
      | 2.nan values caused due to vehicle loosing
      |  its trackalong ref linear path
      | 3.Obstacle collision
      | 4.Max time limit reached for individual
      | forward simulation
  v_0 : Inport
  delta : Inport  Port=2
  gp : Inport  Port=3
  Bus Creator1 : BusCreator  Inputs=8
  Bus Creator2 : BusCreator  Inputs=4
  Bus Creator3 : BusCreator  Inputs=4
  Bus Creator4 : BusCreator  Inputs=2
  Bus Creator6 : BusCreator  Inputs=4
  Bus Selector : BusSelector  OutputSignals=vel_drive_x  OutputAsBus=on
  Bus Selector1 : BusSelector  OutputSignals=vel_drive_y  OutputAsBus=on
  Bus Selector2 : BusSelector  OutputSignals=yawrate_trac  OutputAsBus=on
  Bus Selector3 : BusSelector  OutputSignals=yawrate_semi  OutputAsBus=on
  Data Store Read1 : DataStoreRead  DataStoreName=IC_x0
  Data Store Read2 : DataStoreRead  DataStoreName=IC_y0
  Data Store Read3 : DataStoreRead  DataStoreName=IC_theta0
  Data Store Read4 : DataStoreRead  DataStoreName=IC_theta1
  Data Store Write1 : DataStoreWrite  DataStoreName=itervar1
  Discrete-Time Integrator : DiscreteIntegrator  InitialConditionSource=external  InitialCondition=IC_x0  SampleTime=-1  ICPrevOutput=DiscIntNeverNeededParam  ICPrevScaledInput=DiscIntNeverNeededParam
  Discrete-Time Integrator1 : DiscreteIntegrator  InitialConditionSource=external  InitialCondition=IC_y0  SampleTime=-1  ICPrevOutput=DiscIntNeverNeededParam  ICPrevScaledInput=DiscIntNeverNeededParam
  Discrete-Time Integrator2 : DiscreteIntegrator  InitialConditionSource=external  InitialCondition=IC_theta0  SampleTime=-1  ICPrevOutput=DiscIntNeverNeededParam  ICPrevScaledInput=DiscIntNeverNeededParam
  Discrete-Time Integrator3 : DiscreteIntegrator  InitialConditionSource=external  InitialCondition=IC_theta1  SampleTime=-1  ICPrevOutput=DiscIntNeverNeededParam  ICPrevScaledInput=DiscIntNeverNeededParam
  KM function : MATLAB Function  TreatAsAtomicUnit=on
  Subsystem : Subsystem
  data_bus : Outport  VectorParamsAs1DForOutWhenUnconnected=off
  wires:
  KM function/9(x_1) -> [x_1]
  KM function/10(y_1) -> [y_1]
  KM function/1(x_0_dot) -> [x_0_dot]
  KM function/3(theta_0_dot) -> [theta_0_dot]
  KM function/4(theta_1_dot) -> [theta_1_dot]
  KM function/8(y_1f) -> [y_1f]
  KM function/7(x_1f) -> [x_1f]
  Discrete-Time Integrator/1 -> KM function/1(x_0), [x_0]
  Discrete-Time Integrator1/1 -> KM function/2(y_0), [y_0]
  KM function/11(gamma_1) -> [gamma_1]
  KM function/2(y_0_dot) -> [y_0_dot]
  delta/1 -> [delta], KM function/6(delta)
  Discrete-Time Integrator3/1 -> [theta_1], KM function/4(theta_1)
  KM function/5(x_0f) -> [x_0f]
  KM function/6(y_0f) -> [y_0f]
  v_0/1 -> [v_0], KM function/5(v_0)
  [y_0f] -> Bus Creator1/2  "steer_y"
  [x_1f] -> Bus Creator1/5  "kingpin_x"
  Bus Creator6/1 -> data_bus/1
  [v_1] -> Bus Creator4/2  "velocity_semi"
  [x_0] -> Bus Creator1/3  "drive_x"
  [y_1f] -> Bus Creator1/6  "kingpin_y"
  [x_0f] -> Bus Creator1/1  "steer_x"
  [y_0] -> Bus Creator1/4  "drive_y"
  Bus Creator3/1 -> [SAV_angle]
  [v_0] -> Bus Creator4/1  "velocity_drive"
  [theta_0_dot] -> Bus Creator2/1  "yawrate_trac"
  [theta_1_dot] -> Bus Creator2/2  "yawrate_semi"
  Discrete-Time Integrator2/1 -> [theta_0], KM function/3(theta_0)
  [SAV_rate] -> Bus Selector/1, Bus Selector1/1, Bus Selector3/1, Bus Selector2/1
  Bus Creator2/1 -> [SAV_rate]
  Bus Creator1/1 -> [SAV_pos]
  [delta] -> Bus Creator3/4  "steering_angle"
  [gamma_1] -> Bus Creator3/3  "articulation_angle"
  Bus Creator4/1 -> [SAV_vel]
  [theta_1] -> Bus Creator3/2  "yawangle_semi"
  [SAV_rate] -> Bus Creator6/2  "rate"
  [theta_0] -> Bus Creator3/1  "yawangle_trac"
  [SAV_pos] -> Bus Creator6/1  "pos"
  [SAV_angle] -> Bus Creator6/3  "angle"
  [SAV_vel] -> Bus Creator6/4  "vel"
  Bus Selector3/1 -> Discrete-Time Integrator3/1
  Bus Selector2/1 -> Discrete-Time Integrator2/1
  Bus Selector/1 -> Discrete-Time Integrator/1
  Bus Selector1/1 -> Discrete-Time Integrator1/1
  [y_0_dot] -> Bus Creator2/4  "vel_drive_y"
  [x_0_dot] -> Bus Creator2/3  "vel_drive_x"
  KM function/12(v_1) -> [v_1]
  [x_1] -> Bus Creator1/7  "semi_x"
  [y_1] -> Bus Creator1/8  "semi_y"
  Data Store Read1/1 -> Discrete-Time Integrator/2
  Data Store Read4/1 -> Discrete-Time Integrator3/2
  Data Store Read2/1 -> Discrete-Time Integrator1/2
  Data Store Read3/1 -> Discrete-Time Integrator2/2
  Subsystem/1(Out1) -> Data Store Write1/1
  [theta_1] -> Subsystem/3(theta_1)
  [y_1] -> Subsystem/2(semi_y)
  [x_1] -> Subsystem/1(semi_x)
  [gamma_1] -> Subsystem/4(gamma_1)
  gp/1 -> Subsystem/5(gp)

== system clrrtsf/Chart/propagateorForwardsimulationstage.propagate/Resettable Subsystem/input ==
  data_bus_KM : Inport
  Bus Creator : BusCreator  Inputs=3
  Bus Selector1 : BusSelector  OutputSignals=pos.semi_x,pos.semi_y
  Bus Selector2 : BusSelector  OutputSignals=angle.yawangle_semi
  Constant3 : Constant  Value=0
  Data Store Read : DataStoreRead  DataStoreName=v_0
  Mux1 : Mux  Inputs=3
  Switch : Switch  Criteria=u2 > Threshold
  Out1 : Outport  VectorParamsAs1DForOutWhenUnconnected=off
  wires:
  Data Store Read/1 -> Switch/2, Bus Creator/1  "u_0"
  Bus Creator/1 -> Out1/1
  Constant3/1 -> Mux1/3
  data_bus_KM/1 -> Bus Selector2/1, Bus Selector1/1
  Bus Selector1/1 -> Mux1/1  "<semi_x>"
  Bus Selector1/2 -> Mux1/2  "<semi_y>"
  Mux1/1 -> Switch/1, Switch/3  "semi_pos"
  Switch/1 -> Bus Creator/2  "positions"
  Bus Selector2/1 -> Bus Creator/3  "<yawangle_semi>"

== system clrrtsf/Chart/propagateorForwardsimulationstage.propagate/Subsystem/Subsystem ==
  In1 : Inport
  Data Store Write : DataStoreWrite  DataStoreName=trans1
  wires:
  In1/1 -> Data Store Write/1

== system clrrtsf/Chart/propagateorForwardsimulationstage.propagate/Subsystem/Subsystem1 ==
  note: assigning vehicle final co-ordinates,orientation,
      | and respective reference sample point co-ordinates
      | after individual forward simulation
  gp : Inport
  Data Store Read : DataStoreRead  DataStoreName=veh_path
  Data Store Write1 : DataStoreWrite  DataStoreName=nodevalues
  MATLAB Function : MATLAB Function  TreatAsAtomicUnit=on
  wires:
  Data Store Read/1 -> MATLAB Function/1(veh_path)
  MATLAB Function/1(y) -> Data Store Write1/1
  gp/1 -> MATLAB Function/2(gp)

== system clrrtsf/Chart/stage1.f/For Iterator Subsystem/Subsystem ==
  In2 : Inport
  s : Inport  Port=2
  Enable : EnablePort  StatesWhenEnabling=reset
  2-D Lookup Table : Lookup_n-D  BreakpointsForDimension1=xx  BreakpointsForDimension2=yy  BeginIndexSearchUsingPreviousIndexResult=on  Table=Zf  InternalRulePriority=Speed  RndMeth=Simplest  InputSameDT=on
  Demux : Demux  Outputs=2
  MATLAB Function1 : MATLAB Function  TreatAsAtomicUnit=on
  cost : Outport
  wires:
  MATLAB Function1/1(localco_ord) -> Demux/1
  In2/1 -> MATLAB Function1/1(Nn3)
  Demux/2 -> 2-D Lookup Table/2
  s/1 -> MATLAB Function1/2(s)
  Demux/1 -> 2-D Lookup Table/1
  2-D Lookup Table/1 -> cost/1

== system clrrtsf/Chart/stage1.f/For Iterator Subsystem/Subsystem1 ==
  In2 : Inport
  s : Inport  Port=2
  Enable : EnablePort  StatesWhenEnabling=reset
  2-D Lookup Table : Lookup_n-D  BreakpointsForDimension1=xx  BreakpointsForDimension2=yy  BeginIndexSearchUsingPreviousIndexResult=on  Table=Zr  InternalRulePriority=Speed  RndMeth=Simplest  InputSameDT=on
  Demux : Demux  Outputs=2
  MATLAB Function1 : MATLAB Function  TreatAsAtomicUnit=on
  cost : Outport
  wires:
  Demux/1 -> 2-D Lookup Table/1
  s/1 -> MATLAB Function1/2(s)
  Demux/2 -> 2-D Lookup Table/2
  In2/1 -> MATLAB Function1/1(Nn3)
  MATLAB Function1/1(localco_ord) -> Demux/1
  2-D Lookup Table/1 -> cost/1

== system clrrtsf/Chart/stage1.f_/For Iterator Subsystem/Subsystem ==
  In2 : Inport
  s : Inport  Port=2
  Enable : EnablePort  StatesWhenEnabling=reset
  2-D Lookup Table : Lookup_n-D  BreakpointsForDimension1=xx  BreakpointsForDimension2=yy  BeginIndexSearchUsingPreviousIndexResult=on  Table=Zf  InternalRulePriority=Speed  RndMeth=Simplest  InputSameDT=on
  Demux : Demux  Outputs=2
  MATLAB Function1 : MATLAB Function  TreatAsAtomicUnit=on
  cost : Outport
  wires:
  MATLAB Function1/1(localco_ord) -> Demux/1
  In2/1 -> MATLAB Function1/1(Nn3)
  Demux/2 -> 2-D Lookup Table/2
  s/1 -> MATLAB Function1/2(s)
  Demux/1 -> 2-D Lookup Table/1
  2-D Lookup Table/1 -> cost/1

== system clrrtsf/Chart/stage1.f_/For Iterator Subsystem/Subsystem1 ==
  In2 : Inport
  s : Inport  Port=2
  Enable : EnablePort  StatesWhenEnabling=reset
  2-D Lookup Table : Lookup_n-D  BreakpointsForDimension1=xx  BreakpointsForDimension2=yy  BeginIndexSearchUsingPreviousIndexResult=on  Table=Zr  InternalRulePriority=Speed  RndMeth=Simplest  InputSameDT=on
  Demux : Demux  Outputs=2
  MATLAB Function1 : MATLAB Function  TreatAsAtomicUnit=on
  cost : Outport
  wires:
  Demux/1 -> 2-D Lookup Table/1
  s/1 -> MATLAB Function1/2(s)
  Demux/2 -> 2-D Lookup Table/2
  In2/1 -> MATLAB Function1/1(Nn3)
  MATLAB Function1/1(localco_ord) -> Demux/1
  2-D Lookup Table/1 -> cost/1

== system clrrtsf/Chart/propagateorForwardsimulationstage.propagate/Resettable Subsystem/Controller/Differentiator//filter ==
  In1 : Inport
  Discrete-Time Integrator : DiscreteIntegrator  SampleTime=-1  ICPrevOutput=DiscIntNeverNeededParam  ICPrevScaledInput=DiscIntNeverNeededParam
  Discrete-Time Integrator1 : DiscreteIntegrator  SampleTime=-1  ICPrevOutput=DiscIntNeverNeededParam  ICPrevScaledInput=DiscIntNeverNeededParam
  Gain : Gain  Gain=c  SaturateOnIntegerOverflow=on  OutDataTypeStr=Inherit: Same as input  ParamDataTypeStr=Inherit: Same as input
  Gain1 : Gain  Gain=2*sqrt(c)  SaturateOnIntegerOverflow=on  OutDataTypeStr=Inherit: Same as input  ParamDataTypeStr=Inherit: Same as input
  Sum1 : Sum  Inputs=-+|  SaturateOnIntegerOverflow=on
  Sum2 : Sum  Inputs=-+|  SaturateOnIntegerOverflow=on
  To Workspace : ToWorkspace  VariableName=steering_rate  SampleTime=-1
  To Workspace1 : ToWorkspace  VariableName=steering_acceleration  SampleTime=-1
  Out1 : Outport
  wires:
  Discrete-Time Integrator1/1 -> Discrete-Time Integrator/1, To Workspace/1, Gain1/1
  Discrete-Time Integrator/1 -> Out1/1, Sum2/1
  Sum1/1 -> Discrete-Time Integrator1/1, To Workspace1/1
  Sum2/1 -> Gain/1
  In1/1 -> Sum2/2
  Gain1/1 -> Sum1/1
  Gain/1 -> Sum1/2

== system clrrtsf/Chart/propagateorForwardsimulationstage.propagate/Resettable Subsystem/Controller/purepursuit_contrroller ==
  note: trailer wheel base
  note: Intersection point
      | btwn ref line and lookahead circle
  driveaxle : Inport
  yawangle_semi : Inport  Port=2
  gp : Inport  Port=3
  Nn_ : Inport  Port=4
  Data Store Read : DataStoreRead  DataStoreName=tn  DataStoreElements=tn(:,1:3)
  Data Store Read1 : DataStoreRead  DataStoreName=L_1f
  Data Store Write : DataStoreWrite  DataStoreName=ip
  Gain2 : Gain  Gain=[1 1 0]
  Look ahead radius at semi-trailer axel mid point : Constant  Value=LD
  func to calculate points of intersections : MATLAB Function  TreatAsAtomicUnit=on
  pure pursuit control law : MATLAB Function  TreatAsAtomicUnit=on
  steeringangle : Outport  VectorParamsAs1DForOutWhenUnconnected=off
  wires:
  Data Store Read1/1 -> pure pursuit control law/3(L_1f)
  func to calculate points of intersections/1(P) -> pure pursuit control law/1(P)
  pure pursuit control law/1(ip) -> Data Store Write/1
  Look ahead radius at semi-trailer axel mid point/1 -> func to calculate points of intersections/4(R), pure pursuit control law/6(R)
  pure pursuit control law/2(alpha) -> steeringangle/1
  gp/1 -> func to calculate points of intersections/1(gp), pure pursuit control law/2(gp)
  Gain2/1 -> func to calculate points of intersections/5(pos), pure pursuit control law/5(pos)  "reaction point (x,y)"
  driveaxle/1 -> Gain2/1
  yawangle_semi/1 -> pure pursuit control law/4(yawangle_semi)
  Nn_/1 -> func to calculate points of intersections/2(Nn_)
  Data Store Read/1 -> func to calculate points of intersections/3(tn)
